simulink model "lcm"  (R2012b)
settings: Solver=ode45  StartTime=0.0  StopTime=inf  RelTol=1e-3
values from neighbouring files (symbols this model uses):
  Cb = 10e-9    (= 1e-08)    [LmatcherCalculations1.m]
  Clb = 2e-9    (= 2e-09)    [LmatcherCalculations1.m]
  Lb = Xlb./(2.*pi.*Freq)    [LmatcherCalculations1.m]
  LL = XL./(2.*pi.*Freq)    [LmatcherCalculations1.m]
  Ls = Xs./(2.*pi.*Freq)    [LmatcherCalculations1.m]
  RL = [20 20]    [LmatcherCalculations1.m]
libraries: nesl_utility x16, fl_lib x13, elec_lib x5, simulink x4
settings Model: Creator=p  LastModifiedBy=p

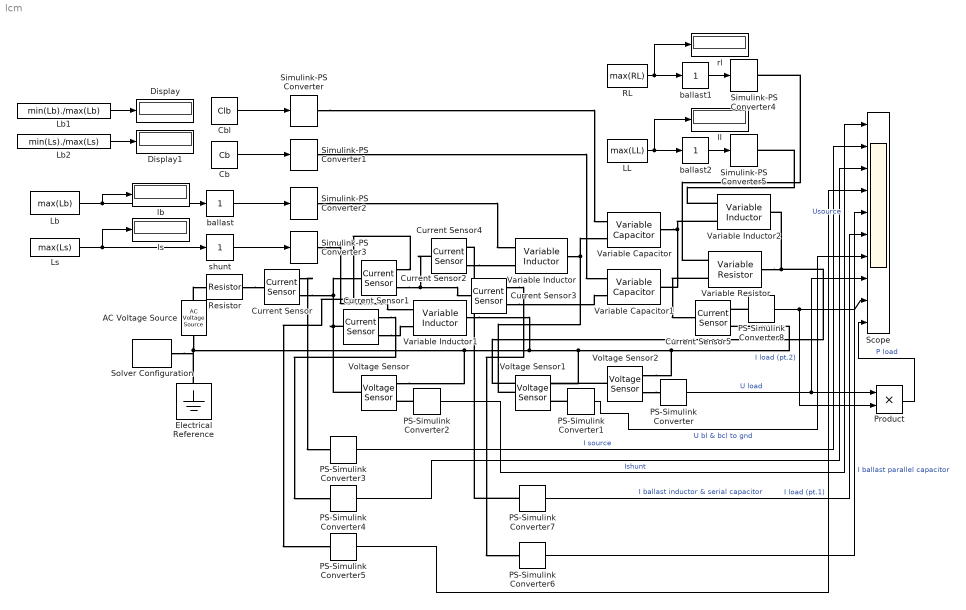
== system lcm ==
  AC Voltage Source : fl_lib/Electrical/Electrical Sources/AC Voltage Source  amp=sqrt(2)*sqrt(500*50).*2 V  shift=0 rad  omega=2e6 Hz  i_Log=off  v_Log=off  LocalVarNames=|i|v  LocalVarDescs=|i|v  LocalVarLogging=[0 0]
  Cb : Constant  Value=Cb  SampleTime=-1
  Cbl : Constant  Value=Clb  SampleTime=-1
  Current Sensor{,1..5} (6 alike) : fl_lib/Electrical/Electrical Sensors/Current Sensor  i1_Log=off  v1_Log=off  LocalVarNames=|i1|v1  LocalVarDescs=|i1|v1  LocalVarLogging=[0 0]
  Display : Display
  Display1 : Display
  Electrical Reference : fl_lib/Electrical/Electrical Elements/Electrical Reference  i_Log=off  LocalVarNames=|i  LocalVarDescs=|i  LocalVarLogging=0
  LL : Constant  Value=max(LL)  SampleTime=-1
  Lb : Constant  Value=max(Lb)  SampleTime=-1
  Lb1 : Constant  Value=min(Lb)./max(Lb)  SampleTime=-1
  Lb2 : Constant  Value=min(Ls)./max(Ls)  SampleTime=-1
  Ls : Constant  Value=max(Ls)  SampleTime=-1
  PS-Simulink Converter{,1..8} (9 alike) : nesl_utility/PS-Simulink Converter  PhysicalDomain=network_engine_domain  LeftPortType=input  RightPortType=output  SubClassName=ps_output  PseudoPeriodic=off  Frequencies=[]  Unit=1  AffineConversion=off
  Product : Product  RndMeth=Zero
  RL : Constant  Value=max(RL)  SampleTime=-1
  Resistor : fl_lib/Electrical/Electrical Elements/Resistor  R=50 Ohm  i_Log=off  v_Log=off  LocalVarNames=|i|v  LocalVarDescs=|i|v  LocalVarLogging=[0 0]
  Scope : Scope  NumInputPorts=10
      settings: ShowLegends=on  TimeRange=1e-06  YMin=-300~-5~-30~-30~-40~-40~-3000~-150~-7.5~0  YMax=300~5~30~30~40~40~3000~150~7.5~1100
  Simulink-PS Converter{,1..5} (6 alike) : nesl_utility/Simulink-PS Converter  PhysicalDomain=network_engine_domain  LeftPortType=input  RightPortType=output  SubClassName=ps_input  PseudoPeriodic=off  Frequencies=[]  NoiseDistribution=none  NoiseParameters=[]  Unit=1  AffineConversion=off  InputFilterTimeConstant=.001  UdotUserProvided=[]  SimscapeFilterOrder=1  InputFiltering=off
  Solver Configuration : nesl_utility/Solver Configuration  PhysicalDomain=network_engine_domain  LeftPortType=input  RightPortType=generic  SubClassName=solver  Accelerate=off  Profile=off  UseLocalSampling=off  FrequencyDomain=off  Tones=[]  Harmonics=[]  UseCCode=off  SimulateNoise=off  EnableSwitchedLinearOptims=on  DoDC=off  ResidualTolerance=1e-9  UseLocalSolver=off  LocalSolverChoice=NE_BACKWARD_EULER_ADVANCER  LocalSolverSampleTime=.001  DoFixedCost=off  MaxNonlinIter=3  MaxModeIter=2  LinearAlgebra=Sparse  DelaysMemoryBudget=1024
  Variable Capacitor : elec_lib/Passive Devices/Variable Capacitor  prm=1  Cmin=1e-12 F  r=1e-9 Ohm  v0=0 V  q0=0 c  LocalVarLogging=[]
  Variable Capacitor1 : elec_lib/Passive Devices/Variable Capacitor  prm=1  Cmin=1e-12 F  r=1e-9 Ohm  v0=0 V  q0=0 c  LocalVarLogging=[]
  Variable Inductor : elec_lib/Passive Devices/Variable Inductor  prm=1  Lmin=1e-12 H  g=1e-9 1/Ohm  i0=0 A  phi0=0 Wb  LocalVarLogging=[]
  Variable Inductor1 : elec_lib/Passive Devices/Variable Inductor  prm=1  Lmin=1e-12 H  g=1e-9 1/Ohm  i0=0 A  phi0=0 Wb  LocalVarLogging=[]
  Variable Inductor2 : elec_lib/Passive Devices/Variable Inductor  prm=1  Lmin=1e-12 H  g=1e-9 1/Ohm  i0=0 A  phi0=0 Wb  LocalVarLogging=[]
  Variable Resistor : fl_lib/Electrical/Electrical Elements/Variable Resistor  Rmin=0 Ohm  i_Log=off  v_Log=off  LocalVarNames=|i|v  LocalVarDescs=|i|v  LocalVarLogging=[0 0]
  Voltage Sensor : fl_lib/Electrical/Electrical Sensors/Voltage Sensor  i1_Log=off  v1_Log=off  LocalVarNames=|i1|v1  LocalVarDescs=|i1|v1  LocalVarLogging=[0 0]
  Voltage Sensor1 : fl_lib/Electrical/Electrical Sensors/Voltage Sensor  i1_Log=off  v1_Log=off  LocalVarNames=|i1|v1  LocalVarDescs=|i1|v1  LocalVarLogging=[0 0]
  Voltage Sensor2 : fl_lib/Electrical/Electrical Sensors/Voltage Sensor  i1_Log=off  v1_Log=off  LocalVarNames=|i1|v1  LocalVarDescs=|i1|v1  LocalVarLogging=[0 0]
  ballast : simulink/Math Operations/Slider Gain  low=0.8  gain=1  high=1
  ballast1 : simulink/Math Operations/Slider Gain  low=0.1  gain=1  high=10
  ballast2 : simulink/Math Operations/Slider Gain  low=0.1  gain=1  high=10
  lb : Display
  ll : Display
  ls : Display
  rl : Display
  shunt : simulink/Math Operations/Slider Gain  low=0.1  gain=1  high=1
  wires:
  Cbl/1 -> Simulink-PS Converter/1
  Cb/1 -> Simulink-PS Converter1/1
  Lb/1 -> lb/1, ballast/1
  Ls/1 -> ls/1, shunt/1
  PS-Simulink Converter2/1 -> Scope/1  "Usource"
  PS-Simulink Converter3/1 -> Scope/2  "I source"
  PS-Simulink Converter4/1 -> Scope/3  "Ishunt"
  PS-Simulink Converter5/1 -> Scope/4  "I load (pt.1)"
  PS-Simulink Converter6/1 -> Scope/5  "I ballast parallel capacitor"
  PS-Simulink Converter7/1 -> Scope/6  "I ballast inductor & serial capacitor"
  PS-Simulink Converter1/1 -> Scope/7  "U bl & bcl to gnd"
  PS-Simulink Converter/1 -> Product/1, Scope/8  "U load"
  PS-Simulink Converter8/1 -> Scope/9, Product/2  "I load (pt.2)"
  ballast/1 -> Simulink-PS Converter2/1
  shunt/1 -> Simulink-PS Converter3/1
  Lb1/1 -> Display/1
  Lb2/1 -> Display1/1
  Product/1 -> Scope/10  "P load"
  RL/1 -> rl/1, ballast1/1
  ballast1/1 -> Simulink-PS Converter4/1
  LL/1 -> ll/1, ballast2/1
  ballast2/1 -> Simulink-PS Converter5/1
  connections:
  Variable Capacitor/RConn1 -- Variable Capacitor1/RConn1 -- Variable Inductor2/LConn2
  Variable Inductor/RConn1 -- Voltage Sensor1/LConn1 -- Variable Capacitor/LConn2
  AC Voltage Source/LConn1 -- Resistor/LConn1
  Current Sensor2/RConn2 -- Current Sensor4/LConn1 -- Current Sensor3/LConn1
  Simulink-PS Converter/RConn1 -- Variable Capacitor/LConn1
  Simulink-PS Converter1/RConn1 -- Variable Capacitor1/LConn1
  Simulink-PS Converter2/RConn1 -- Variable Inductor/LConn1
  Simulink-PS Converter3/RConn1 -- Variable Inductor1/LConn1
  Variable Resistor/LConn1 -- Simulink-PS Converter4/RConn1
  Voltage Sensor2/RConn1 -- PS-Simulink Converter/LConn1
  PS-Simulink Converter1/LConn1 -- Voltage Sensor1/RConn1
  PS-Simulink Converter2/LConn1 -- Voltage Sensor/RConn1
  Resistor/RConn1 -- Current Sensor/LConn1
  Current Sensor/RConn1 -- PS-Simulink Converter3/LConn1
  Current Sensor1/RConn2 -- Variable Inductor1/LConn2
  Current Sensor1/RConn1 -- PS-Simulink Converter4/LConn1
  Current Sensor1/LConn1 -- Current Sensor/RConn2 -- Current Sensor2/LConn1 -- Voltage Sensor/LConn1
  Current Sensor2/RConn1 -- PS-Simulink Converter5/LConn1
  Current Sensor3/RConn2 -- Variable Capacitor1/LConn2
  Current Sensor3/RConn1 -- PS-Simulink Converter6/LConn1
  Current Sensor4/RConn2 -- Variable Inductor/LConn2
  PS-Simulink Converter7/LConn1 -- Current Sensor4/RConn1
  PS-Simulink Converter8/LConn1 -- Current Sensor5/RConn1
  Voltage Sensor/RConn2 -- Current Sensor5/RConn2 -- Voltage Sensor2/RConn2 -- Voltage Sensor1/RConn2 -- Variable Inductor1/RConn1 -- Electrical Reference/LConn1 -- Solver Configuration/RConn1 -- AC Voltage Source/RConn1
  Variable Resistor/RConn1 -- Variable Inductor2/RConn1 -- Voltage Sensor2/LConn1
  Variable Inductor2/LConn1 -- Simulink-PS Converter5/RConn1
  Variable Resistor/LConn2 -- Current Sensor5/LConn1
